simulink model "SinglePhasePWMInverter"  (R2024b)
settings: Solver=FixedStepDiscrete  StartTime=0.0  StopTime=0.07  FixedStep=5e-6  RelTol=1e-4  EnableMultiTasking=on
PreLoadFcn:
  | Ts=5e-6;
InitFcn:
  | Ts=5e-6;
libraries: spsGroundLib x6, spsDCVoltageSourceLib x3, spsSeriesRLCBranchLib x2, spsCurrentMeasurementLib x2, spsVoltageMeasurementLib x2, spsPWMGenerator2LevelLib x2, spsFullBridgeConverterLib x1, spsHalfBridgeConverterLib x1, spspowerguiLib x1
settings Model: Creator=The MathWorks, Inc.  LastModifiedBy=The MathWorks, Inc.
settings SolverCC: AlgebraicLoopSolver=TrustRegion  SolverResetMethod=Robust
settings DataIOCC: SaveOutput=off  SignalLogging=off  DSMLogging=off  SaveTime=off  ReturnWorkspaceOutputs=off
settings OptimizationCC: LifeSpan=inf
settings DebuggingCC: ReadBeforeWriteMsg=DisableAll  WriteAfterWriteMsg=DisableAll  WriteAfterReadMsg=DisableAll  MultiTaskDSMMsg=none  UnconnectedInputMsg=warning  UnconnectedOutputMsg=warning  UnconnectedLineMsg=warning  SFUnexpectedBacktrackingDiag=warning  SFNoUnconditionalDefaultTransitionDiag=warning  SFExecutionAtInitializationDiag=none  ArithmeticOperatorsInVariantConditions=warning
settings ModelReferenceCC: UpdateModelReferenceTargets=IfOutOfDate  EnableRefExpFcnMdlSchedulingChecks=on
settings SFSimCC: SFSimEcho=off  SimUseLocalCustomCode=off  CustomCodeUndefinedFunction=UseInterfaceOnly
settings RTWCC: RTWUseLocalCustomCode=off  GPUComputeCapability=3.5
settings CodeAppCC: StateflowObjectComments=on
settings GRTTargetCC: TargetLangStandard=C89/C90 (ANSI)
settings ConfigComp: CovMetricSettings=dw  CovSaveCumulativeToWorkspaceVar=on  CovSaveSingleToWorkspaceVar=on  CovExternalEMLEnable=off
settings SimscapeCC: SimscapeNormalizeSystem=off  SimscapeNominalValues={1, 'bar'; 1, 'cm^3/s'; 1, 'bar*kg/s'; 1, 'kJ/kg'; 1, 'kW'; }

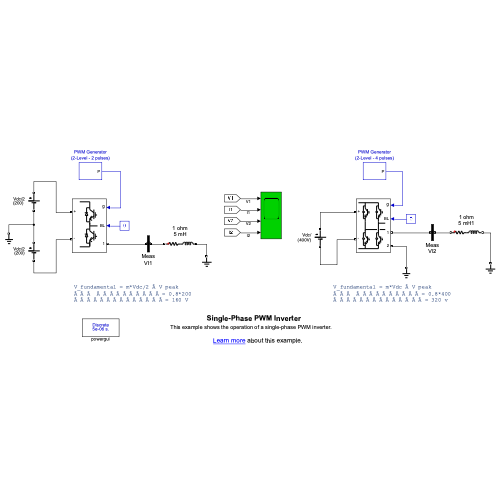
[thumbnail: Simulink's stored preview of the top-level diagram]
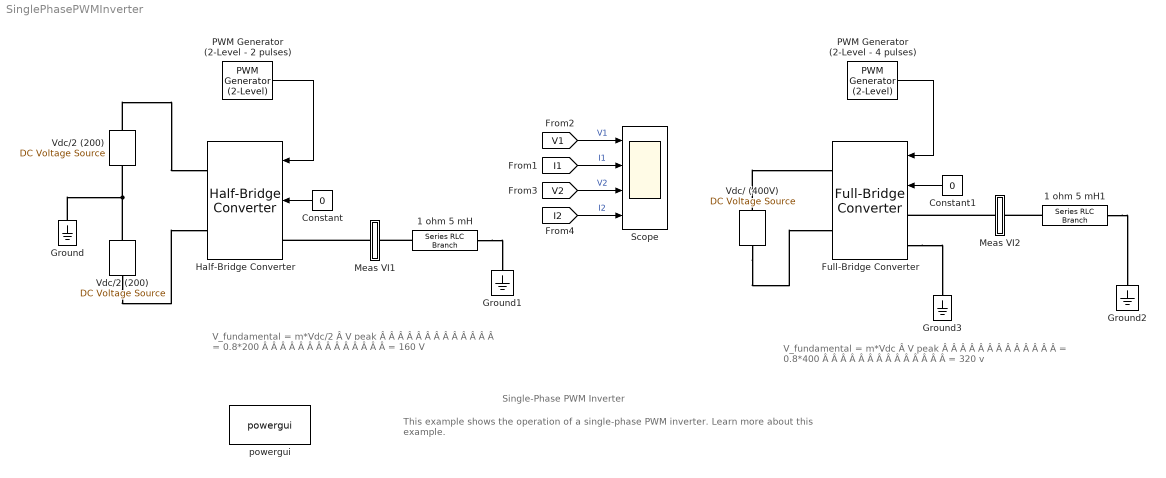
== system SinglePhasePWMInverter ==
  note: V_fundamental = m*Vdc/2 Â V peak
      | Â Â Â Â Â Â Â Â Â Â Â Â Â = 0.8*200
      | Â Â Â Â Â Â Â Â Â Â Â Â Â Â = 160 V
  note: Single-Phase PWM Inverter
  note: This example shows the operation of a single-phase PWM inverter.
      |
      | Learn more about this example.
  note: V_fundamental = m*Vdc Â V peak
      | Â Â Â Â Â Â Â Â Â Â Â Â Â = 0.8*400
      | Â Â Â Â Â Â Â Â Â Â Â Â Â Â = 320 v
  1 ohm 5 mH : spsSeriesRLCBranchLib/Series RLC Branch  LConnTagsString=__new0  RConnTagsString=__new0  BranchType=RL  Resistance=1  Inductance=5e-3  SetiL0=off  InitialCurrent=0  Capacitance=400e-6  Setx0=off  InitialVoltage=0  Measurements=None
  1 ohm 5 mH1 : spsSeriesRLCBranchLib/Series RLC Branch  LConnTagsString=__new0  RConnTagsString=__new0  BranchType=RL  Resistance=1  Inductance=5e-3  SetiL0=off  InitialCurrent=0  Capacitance=400e-6  Setx0=off  InitialVoltage=0  Measurements=None
  Constant : Constant  Value=0
  Constant1 : Constant  Value=0
  Full-Bridge Converter : spsFullBridgeConverterLib/Full-Bridge Converter  ModelType=Switching devices  Ron=1e-3  Rs=1e6  Cs=inf  Vforward=[0,0]  Ron_Diode=1e-3  Rs_Diode=1e6  Cs_Diode=inf  Vf_Diode=1e-3  Rs_CurrentSource=inf  Ron_ACsource=1e-3
      settings: LibrarySourceBlock=sps_lib/Power Electronics/Full-Bridge Converter
  Ground{,1..3} (4 alike) : spsGroundLib/Ground  LConnTagsString=a
  Half-Bridge Converter : spsHalfBridgeConverterLib/Half-Bridge Converter  ModelType=Switching devices  Ron=1e-3  Rs=1e6  Cs=inf  Vforward=[0,0]  Ron_Diode=1e-3  Rs_Diode=1e6  Cs_Diode=inf  Vf_Diode=1e-3  Rs_CurrentSource=inf  Ron_ACsource=1e-3
      settings: LibrarySourceBlock=sps_lib/Power Electronics/Half-Bridge Converter
  Meas VI1 : Subsystem
  Meas VI2 : Subsystem
  PWM Generator (2-Level - 2 pulses) : spsPWMGenerator2LevelLib/PWM Generator (2-Level)  ModulatorType=Single-phase half-bridge (2 pulses)  ModulatorMode=Unsynchronized  Fc=27*60  Pc=90  nF=27  MinMax="[ -1  1 ]"  SamplingTechnique=Natural  ModulatingSignals=on  m=0.8  Freq=60  Phase=0  Ts=5e-6  ShowCarrierOutport=off
  PWM Generator (2-Level - 4 pulses) : spsPWMGenerator2LevelLib/PWM Generator (2-Level)  ModulatorType=Single-phase full-bridge (4 pulses)  ModulatorMode=Unsynchronized  Fc=27*60  Pc=90  nF=27  MinMax="[ -1  1 ]"  SamplingTechnique=Natural  ModulatingSignals=on  m=0.8  Freq=60  Phase=0  Ts=5e-6  ShowCarrierOutport=off
  Scope : Scope  NumInputPorts=4
  Vdc/ (400V) : spsDCVoltageSourceLib/DC Voltage Source  Amplitude=400  Measurements=None
  Vdc/2 (200) : spsDCVoltageSourceLib/DC Voltage Source  Amplitude=200  Measurements=None
  "Vdc/2 (200) " : spsDCVoltageSourceLib/DC Voltage Source  Amplitude=200  Measurements=None
  powergui : spspowerguiLib/powergui  Priority=1  SimulationMode=Discrete  SampleTime=5e-6  frequency=60  Iterations=50  frequencyindice=0  Pbase=100e6  ErrMax=1e-4  UnitsV=kV  UnitsW=MW  buscounter=0  FunctionMessages=off  echomessages=off  EnableUseOfTLC=off  CurrentSourceSwitches=off  DisableSnubberDevices=off  DisableRonSwitches=off  DisableVfSwitches=off  DisplayEquations=off  AutomaticDiscreteSolvers=off  SolverType=Tustin/Backward Euler (TBE)  Interpol=off  ExternalGateDelay=off  methode=off  Ts=100  x0status=blocks  SPID=off  SwTol=0  HookPort=off  NonlinearTolerance=1e-4  nMaxIteration=100  ContinueOnMaxIteration=off  RestoreLinks=warning  ResistiveCurrentMeasurement=off  Frange=[0:2:500]  Ylog=off  Xlog=on  ShowGrid=off  save=off  variable=ZData  structure=ScopeDataForFFT  ZoomFFT=off  StartTime=0.07-2/60  cycles=2  DisplayStyle=1  fundamental=60  FreqAxis=off  MaxFrequency=5000  frequencyindicesteady=1  RmsSteady=1  display=off
  wires:
  [V1] -> Scope/1  "V1"
  PWM Generator (2-Level - 2 pulses)/1 -> Half-Bridge Converter/1
  Constant/1 -> Half-Bridge Converter/2
  PWM Generator (2-Level - 4 pulses)/1 -> Full-Bridge Converter/1
  Constant1/1 -> Full-Bridge Converter/2
  [V2] -> Scope/3  "V2"
  [I2] -> Scope/4  "I2"
  [I1] -> Scope/2  "I1"
  connections:
  Vdc/2 (200)/RConn1 -- Ground/LConn1 -- "Vdc/2 (200) "/LConn1
  "Vdc/2 (200) "/RConn1 -- Half-Bridge Converter/RConn1
  Vdc/2 (200)/LConn1 -- Half-Bridge Converter/RConn2
  Meas VI1/LConn1 -- Half-Bridge Converter/LConn1
  1 ohm 5 mH/LConn1 -- Meas VI1/RConn1
  1 ohm 5 mH/RConn1 -- Ground1/LConn1
  Meas VI2/LConn1 -- Full-Bridge Converter/LConn1
  1 ohm 5 mH1/RConn1 -- Ground2/LConn1
  1 ohm 5 mH1/LConn1 -- Meas VI2/RConn1
  Vdc/ (400V)/RConn1 -- Full-Bridge Converter/RConn1
  Vdc/ (400V)/LConn1 -- Full-Bridge Converter/RConn2
  Full-Bridge Converter/LConn2 -- Ground3/LConn1

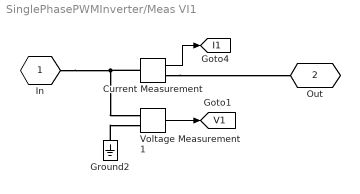
== system SinglePhasePWMInverter/Meas VI1 ==
  Current Measurement : spsCurrentMeasurementLib/Current Measurement  PhasorSimulation=off  OutputType=Complex  PSBequivalent=0
  Ground2 : spsGroundLib/Ground  LConnTagsString=a
  Voltage Measurement1 : spsVoltageMeasurementLib/Voltage Measurement  Tag=PoWeRsYsTeMmEaSuReMeNt  PhasorSimulation=off  OutputType=Magnitude  PSBequivalent=0
  In : PMIOPort  Tag=PMCPort  Side=Left
  Out : PMIOPort  Tag=PMCPort  Port=2  Side=Right
  tag scope: I1=global, V1=global
  wires:
  Current Measurement/1 -> [I1]
  Voltage Measurement1/1 -> [V1]
  connections:
  Ground2/LConn1 -- Voltage Measurement1/LConn2
  In/RConn1 -- Current Measurement/LConn1 -- Voltage Measurement1/LConn1
  Current Measurement/RConn1 -- Out/RConn1

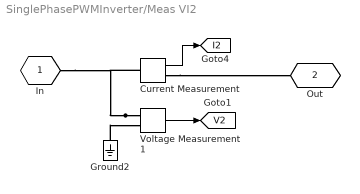
== system SinglePhasePWMInverter/Meas VI2 ==
  Current Measurement : spsCurrentMeasurementLib/Current Measurement  PhasorSimulation=off  OutputType=Complex  PSBequivalent=0
  Ground2 : spsGroundLib/Ground  LConnTagsString=a
  Voltage Measurement1 : spsVoltageMeasurementLib/Voltage Measurement  Tag=PoWeRsYsTeMmEaSuReMeNt  PhasorSimulation=off  OutputType=Magnitude  PSBequivalent=0
  In : PMIOPort  Tag=PMCPort  Side=Left
  Out : PMIOPort  Tag=PMCPort  Port=2  Side=Right
  tag scope: I2=global, V2=global
  wires:
  Voltage Measurement1/1 -> [V2]
  Current Measurement/1 -> [I2]
  connections:
  Current Measurement/RConn1 -- Out/RConn1
  Voltage Measurement1/LConn1 -- Current Measurement/LConn1 -- In/RConn1
  Ground2/LConn1 -- Voltage Measurement1/LConn2
